simulink model "SimulationANTSMC"  (R2020b)
settings: Solver=ode3  StartTime=0.0  StopTime=100  FixedStep=0.001  RelTol=1e-6  EnableMultiTasking=on
model workspace (MAT data in the model file):
  time = 1
values from neighbouring files (symbols this model uses):
  beta = 2*x(3)/(1+x(3))    [GA_init.m]
  epstar = x(9)    [GA_init.m]
  g0 = x(5)    [GA_init.m]
  g1 = x(6)    [GA_init.m]
  g2 = x(7)    [GA_init.m]
  g3 = x(8)    [GA_init.m]
  gamma = x(3)    [GA_init.m]
  kappa = x(11)    [GA_init.m]
  landa = x(1)    [GA_init.m]
  nu = x(2)    [GA_init.m]
  vu = x(4)    [GA_init.m]
(part 9 of 18)

== matlab function SimulationANTSMC/Subsystem/System Dynamics ==
  data: disturbance output; u input; thetadot input; theta input; t input; y output
function [disturbance,y] = fcn(u,thetadot,theta,t)

theta1=theta(1);
theta2=theta(2);
theta3=theta(3);
theta4=theta(4);
theta5=theta(5);
theta6=theta(6);

thetadot1=thetadot(1);
thetadot2=thetadot(2);
thetadot3=thetadot(3);
thetadot4=thetadot(4);
thetadot5=thetadot(5);
thetadot6=thetadot(6);


MM =[ 0.1*cos(theta2 + theta3)^2 + (0.6*cos(theta2)*cos(theta4)*cos(theta6) + 0.2*cos(theta2)*cos(theta5)*sin(theta3) + 0.2*cos(theta3)*cos(theta5)*sin(theta2) + 1.5*cos(theta2)*cos(theta3)*cos(theta4)*cos(theta6) + 0.2*cos(theta2)*cos(theta3)*cos(theta4)*sin(theta5) + 1.4*cos(theta2)*cos(theta3)*sin(theta4)*sin(theta6) - 1.5*cos(theta4)*cos(theta6)*sin(theta2)*sin(theta3) + 1.4*cos(theta2)*cos(theta6)*sin(theta3)*sin(theta5) + 1.4*cos(theta3)*cos(theta6)*sin(theta2)*sin(theta5) - 0.6*cos(theta2)*cos(theta5)*sin(theta4)*sin(theta6) - 0.2*cos(theta4)*sin(theta2)*sin(theta3)*sin(theta5) - 1.4*sin(theta2)*sin(theta3)*sin(theta4)*sin(theta6) - 1.4*cos(theta2)*cos(theta3)*cos(theta4)*cos(theta5)*cos(theta6) - 1.5*cos(theta2)*cos(theta3)*cos(theta5)*sin(theta4)*sin(theta6) + 1.4*cos(theta4)*cos(theta5)*cos(theta6)*sin(theta2)*sin(theta3) + 1.5*cos(theta5)*sin(theta2)*sin(theta3)*sin(theta4)*sin(theta6))^2 + 0.101*sin(theta2 + theta3)^2 + (0.2*cos(theta6)*sin(theta2)*sin(theta3)*sin(theta4) - 0.2*cos(theta2)*cos(theta3)*cos(theta6)*sin(theta4) - 1.5*cos(theta2)*cos(theta3)*sin(theta4)*sin(theta5) - 0.6*cos(theta2)*sin(theta4)*sin(theta5) + 0.2*cos(theta2)*sin(theta3)*sin(theta5)*sin(theta6) + 0.2*cos(theta3)*sin(theta2)*sin(theta5)*sin(theta6) + 1.5*sin(theta2)*sin(theta3)*sin(theta4)*sin(theta5) - 0.2*cos(theta2)*cos(theta3)*cos(theta4)*cos(theta5)*sin(theta6) + 0.2*cos(theta4)*cos(theta5)*sin(theta2)*sin(theta3)*sin(theta6))^2 + (0.6*cos(theta2)*cos(theta4) - 1.5*cos(theta4)*sin(theta2)*sin(theta3) + 1.4*cos(theta2)*sin(theta3)*sin(theta5) + 1.4*cos(theta3)*sin(theta2)*sin(theta5) + 1.5*cos(theta2)*cos(theta3)*cos(theta4) + 0.2*cos(theta2)*cos(theta5)*sin(theta3) + 0.2*cos(theta3)*cos(theta5)*sin(theta2) - 1.4*cos(theta2)*cos(theta3)*cos(theta4)*cos(theta5) + 0.2*cos(theta2)*cos(theta3)*cos(theta4)*sin(theta5) + 1.4*cos(theta4)*cos(theta5)*sin(theta2)*sin(theta3) - 0.2*cos(theta4)*sin(theta2)*sin(theta3)*sin(theta5))^2 + (0.0001*cos(theta6)*sin(theta2)*sin(theta3)*sin(theta4) - 0.0001*cos(theta2)*cos(theta3)*cos(theta6)*sin(theta4) + 0.0001*cos(theta2)*sin(theta3)*sin(theta5)*sin(theta6) + 0.0001*cos(theta3)*sin(theta2)*sin(theta5)*sin(theta6) - 0.0001*cos(theta2)*cos(theta3)*cos(theta4)*cos(theta5)*sin(theta6) + 0.0001*cos(theta4)*cos(theta5)*sin(theta2)*sin(theta3)*sin(theta6))*(cos(theta6)*sin(theta2)*sin(theta3)*sin(theta4) - 1.0*cos(theta2)*cos(theta3)*cos(theta6)*sin(theta4) + cos(theta2)*sin(theta3)*sin(theta5)*sin(theta6) + cos(theta3)*sin(theta2)*sin(theta5)*sin(theta6) - 1.0*cos(theta2)*cos(theta3)*cos(theta4)*cos(theta5)*sin(theta6) + cos(theta4)*cos(theta5)*sin(theta2)*sin(theta3)*sin(theta6)) + (0.44721359549995793928183473374626*cos(theta2 + theta3 + 0.46364760900080611621425623146121) - 0.6*cos(theta2))^2 + 0.1*cos(theta2)^2 + 0.14*sin(theta2)^2 + (cos(theta2)*cos(theta5)*sin(theta3) + cos(theta3)*cos(theta5)*sin(theta2) + cos(theta2)*cos(theta3)*cos(theta4)*sin(theta5) - 1.0*cos(theta4)*sin(theta2)*sin(theta3)*sin(theta5))*(0.0001*cos(theta2)*cos(theta5)*sin(theta3) + 0.0001*cos(theta3)*cos(theta5)*sin(theta2) + 0.0001*cos(theta2)*cos(theta3)*cos(theta4)*sin(theta5) - 0.0001*cos(theta4)*sin(theta2)*sin(theta3)*sin(theta5)) + 0.01*sin(theta4)^2*(2.0*cos(theta2)*cos(theta3) + 6.0*cos(theta2)*sin(theta5) - 2.0*sin(theta2)*sin(theta3) - 15.0*sin(theta2)*sin(theta3)*sin(theta5) + 15.0*cos(theta2)*cos(theta3)*sin(theta5))^2 + 0.001*cos(theta2 + theta3)^2*cos(theta4)^2 + 0.01*sin(theta4)^2*(cos(theta2 + theta3) - 6.0*cos(theta2))^2 + 0.0415*cos(theta2 + theta3)^2*sin(theta4)^2 + (0.0005*cos(theta2)*cos(theta5)*sin(theta3) + 0.0005*cos(theta3)*cos(theta5)*sin(theta2) + 0.0005*cos(theta2)*cos(theta3)*cos(theta4)*sin(theta5) - 0.0005*cos(theta4)*sin(theta2)*sin(theta3)*sin(theta5))*(cos(theta2)*cos(theta5)*sin(theta3) + cos(theta3)*cos(theta5)*sin(theta2) + cos(theta2)*cos(theta3)*cos(theta4)*sin(theta5) - 1.0*cos(theta4)*sin(theta2)*sin(theta3)*sin(theta5)) + (0.0005*cos(theta2)*sin(theta3)*sin(theta5) + 0.0005*cos(theta3)*sin(theta2)*sin(theta5) - 0.0005*cos(theta2)*cos(theta3)*cos(theta4)*cos(theta5) + 0.0005*cos(theta4)*cos(theta5)*sin(theta2)*sin(theta3))*(cos(theta2)*sin(theta3)*sin(theta5) + cos(theta3)*sin(theta2)*sin(theta5) - 1.0*cos(theta2)*cos(theta3)*cos(theta4)*cos(theta5) + cos(theta4)*cos(theta5)*sin(theta2)*sin(theta3)) + 0.01*sin(theta4)^2*(6.0*cos(theta2)*cos(theta5) - 14.0*cos(theta2)*cos(theta3) + 14.0*sin(theta2)*sin(theta3) - 15.0*cos(theta5)*sin(theta2)*sin(theta3) + 15.0*cos(theta2)*cos(theta3)*cos(theta5))^2 + (0.6*cos(theta2)*cos(theta4) + 0.2*cos(theta2)*sin(theta3) + 0.2*cos(theta3)*sin(theta2) + 0.1*cos(theta4)*sin(theta2)*sin(theta3) - 0.1*cos(theta2)*cos(theta3)*cos(theta4))^2 + (0.0001*cos(theta2)*cos(theta3)*sin(theta4)*sin(theta6) + 0.0001*cos(theta2)*cos(theta6)*sin(theta3)*sin(theta5) + 0.0001*cos(theta3)*cos(theta6)*sin(theta2)*sin(theta5) - 0.0001*sin(theta2)*sin(theta3)*sin(theta4)*sin(theta6) - 0.0001*cos(theta2)*cos(theta3)*cos(theta4)*cos(theta5)*cos(theta6) + 0.0001*cos(theta4)*cos(theta5)*cos(theta6)*sin(theta2)*sin(theta3))*(cos(theta2)*cos(theta3)*sin(theta4)*sin(theta6) + cos(theta2)*cos(theta6)*sin(theta3)*sin(theta5) + cos(theta3)*cos(theta6)*sin(theta2)*sin(theta5) - 1.0*sin(theta2)*sin(theta3)*sin(theta4)*sin(theta6) - 1.0*cos(theta2)*cos(theta3)*cos(theta4)*cos(theta5)*cos(theta6) + cos(theta4)*cos(theta5)*cos(theta6)*sin(theta2)*sin(theta3)) + (0.6*cos(theta2)*cos(theta4)*sin(theta6) + 1.5*cos(theta2)*cos(theta3)*cos(theta4)*sin(theta6) - 1.4*cos(theta2)*cos(theta3)*cos(theta6)*sin(theta4) + 0.6*cos(theta2)*cos(theta5)*cos(theta6)*sin(theta4) - 1.5*cos(theta4)*sin(theta2)*sin(theta3)*sin(theta6) + 1.4*cos(theta6)*sin(theta2)*sin(theta3)*sin(theta4) + 1.4*cos(theta2)*sin(theta3)*sin(theta5)*sin(theta6) + 1.4*cos(theta3)*sin(theta2)*sin(theta5)*sin(theta6) - 1.4*cos(theta2)*cos(theta3)*cos(theta4)*cos(theta5)*sin(theta6) + 1.5*cos(theta2)*cos(theta3)*cos(theta5)*cos(theta6)*sin(theta4) + 1.4*cos(theta4)*cos(theta5)*sin(theta2)*sin(theta3)*sin(theta6) - 1.5*cos(theta5)*cos(theta6)*sin(theta2)*sin(theta3)*sin(theta4))^2 + 0.1, 0.12*sin(theta2)*sin(theta4) + 0.26*cos(theta2)*sin(theta3)*sin(theta4) + 0.26*cos(theta3)*sin(theta2)*sin(theta4) + 0.12*cos(theta5)*sin(theta2)*sin(theta4) + 0.12*cos(theta4)*sin(theta2)*sin(theta6) + 1.68*sin(theta2)*sin(theta4)*sin(theta5) - 0.56*cos(theta2)*cos(theta5)^2*sin(theta3)*sin(theta4) - 0.56*cos(theta3)*cos(theta5)^2*sin(theta2)*sin(theta4) - 3.92*cos(theta2)*cos(theta3)*cos(theta4)*sin(theta4) + 0.3*cos(theta2)*cos(theta5)*sin(theta3)*sin(theta4) + 0.3*cos(theta3)*cos(theta5)*sin(theta2)*sin(theta4) + 0.3*cos(theta2)*cos(theta4)*sin(theta3)*sin(theta6) + 0.28*cos(theta2)*cos(theta6)*sin(theta3)*sin(theta4) + 0.3*cos(theta3)*cos(theta4)*sin(theta2)*sin(theta6) + 0.28*cos(theta3)*cos(theta6)*sin(theta2)*sin(theta4) + 0.28*cos(theta2)*cos(theta3)*sin(theta5)*sin(theta6) + 0.12*cos(theta5)*cos(theta6)*sin(theta2)*sin(theta4) + 3.92*cos(theta4)*sin(theta2)*sin(theta3)*sin(theta4) + 4.2*cos(theta2)*sin(theta3)*sin(theta4)*sin(theta5) + 4.2*cos(theta3)*sin(theta2)*sin(theta4)*sin(theta5) - 0.28*sin(theta2)*sin(theta3)*sin(theta5)*sin(theta6) + 3.88*cos(theta2)*cos(theta3)*cos(theta4)*cos(theta5)^2*sin(theta4) - 0.04*cos(theta2)*cos(theta3)*cos(theta4)*cos(theta6)^2*sin(theta4) - 0.56*cos(theta2)*cos(theta3)*cos(theta4)^2*sin(theta5)*sin(theta6) - 0.56*cos(theta2)*cos(theta5)^2*cos(theta6)*sin(theta3)*sin(theta4) - 0.56*cos(theta3)*cos(theta5)^2*cos(theta6)*sin(theta2)*sin(theta4) - 3.88*cos(theta4)*cos(theta5)^2*sin(theta2)*sin(theta3)*sin(theta4) + 0.04*cos(theta4)*cos(theta6)^2*sin(theta2)*sin(theta3)*sin(theta4) + 0.56*cos(theta4)^2*sin(theta2)*sin(theta3)*sin(theta5)*sin(theta6) + 0.04*cos(theta2)*cos(theta3)*cos(theta5)*cos(theta6)*sin(theta6) - 0.28*cos(theta2)*cos(theta4)*cos(theta5)*sin(theta3)*sin(theta6) + 0.3*cos(theta2)*cos(theta5)*cos(theta6)*sin(theta3)*sin(theta4) - 0.28*cos(theta3)*cos(theta4)*cos(theta5)*sin(theta2)*sin(theta6) + 0.3*cos(theta3)*cos(theta5)*cos(theta6)*sin(theta2)*sin(theta4) - 3.88*cos(theta2)*cos(theta5)*sin(theta3)*sin(theta4)*sin(theta5) - 3.88*cos(theta3)*cos(theta5)*sin(theta2)*sin(theta4)*sin(theta5) - 0.04*cos(theta5)*cos(theta6)*sin(theta2)*sin(theta3)*sin(theta6) - 0.04*cos(theta2)*cos(theta3)*cos(theta4)*cos(theta5)^2*cos(theta6)^2*sin(theta4) + 0.04*cos(theta4)*cos(theta5)^2*cos(theta6)^2*sin(theta2)*sin(theta3)*sin(theta4) - 0.56*cos(theta2)*cos(theta3)*cos(theta4)*cos(theta5)*sin(theta4)*sin(theta5) + 0.04*cos(theta2)*cos(theta4)*cos(theta6)*sin(theta3)*sin(theta5)*sin(theta6) + 0.04*cos(theta3)*cos(theta4)*cos(theta6)*sin(theta2)*sin(theta5)*sin(theta6) + 0.56*cos(theta4)*cos(theta5)*sin(theta2)*sin(theta3)*sin(theta4)*sin(theta5) - 0.08*cos(theta2)*cos(theta3)*cos(theta4)^2*cos(theta5)*cos(theta6)*sin(theta6) + 0.04*cos(theta2)*cos(theta5)*cos(theta6)^2*sin(theta3)*sin(theta4)*sin(theta5) + 0.04*cos(theta3)*cos(theta5)*cos(theta6)^2*sin(theta2)*sin(theta4)*sin(theta5) + 0.08*cos(theta4)^2*cos(theta5)*cos(theta6)*sin(theta2)*sin(theta3)*sin(theta6) - 0.56*cos(theta2)*cos(theta3)*cos(theta4)*cos(theta5)*cos(theta6)*sin(theta4)*sin(theta5) + 0.56*cos(theta4)*cos(theta5)*cos(theta6)*sin(theta2)*sin(theta3)*sin(theta4)*sin(theta5), 0.26*cos(theta2)*sin(theta3)*sin(theta4) + 0.26*cos(theta3)*sin(theta2)*sin(theta4) - 0.56*cos(theta2)*cos(theta5)^2*sin(theta3)*sin(theta4) - 0.56*cos(theta3)*cos(theta5)^2*sin(theta2)*sin(theta4) - 3.92*cos(theta2)*cos(theta3)*cos(theta4)*sin(theta4) + 0.3*cos(theta2)*cos(theta5)*sin(theta3)*sin(theta4) + 0.3*cos(theta3)*cos(theta5)*sin(theta2)*sin(theta4) + 0.3*cos(theta2)*cos(theta4)*sin(theta3)*sin(theta6) + 0.28*cos(theta2)*cos(theta6)*sin(theta3)*sin(theta4) + 0.3*cos(theta3)*cos(theta4)*sin(theta2)*sin(theta6) + 0.28*cos(theta3)*cos(theta6)*sin(theta2)*sin(theta4) + 0.28*cos(theta2)*cos(theta3)*sin(theta5)*sin(theta6) + 3.92*cos(theta4)*sin(theta2)*sin(theta3)*sin(theta4) + 4.2*cos(theta2)*sin(theta3)*sin(theta4)*sin(theta5) + 4.2*cos(theta3)*sin(theta2)*sin(theta4)*sin(theta5) - 0.28*sin(theta2)*sin(theta3)*sin(theta5)*sin(theta6) + 3.88*cos(theta2)*cos(theta3)*cos(theta4)*cos(theta5)^2*sin(theta4) - 0.04*cos(theta2)*cos(theta3)*cos(theta4)*cos(theta6)^2*sin(theta4) - 0.56*cos(theta2)*cos(theta3)*cos(theta4)^2*sin(theta5)*sin(theta6) - 0.56*cos(theta2)*cos(theta5)^2*cos(theta6)*sin(theta3)*sin(theta4) - 0.56*cos(theta3)*cos(theta5)^2*cos(theta6)*sin(theta2)*sin(theta4) - 3.88*cos(theta4)*cos(theta5)^2*sin(theta2)*sin(theta3)*sin(theta4) + 0.04*cos(theta4)*cos(theta6)^2*sin(theta2)*sin(theta3)*sin(theta4) + 0.56*cos(theta4)^2*sin(theta2)*sin(theta3)*sin(theta5)*sin(theta6) + 0.04*cos(theta2)*cos(theta3)*cos(theta5)*cos(theta6)*sin(theta6) - 0.28*cos(theta2)*cos(theta4)*cos(theta5)*sin(theta3)*sin(theta6) + 0.3*cos(theta2)*cos(theta5)*cos(theta6)*sin(theta3)*sin(theta4) - 0.28*cos(theta3)*cos(theta4)*cos(theta5)*sin(theta2)*sin(theta6) + 0.3*cos(theta3)*cos(theta5)*cos(theta6)*sin(theta2)*sin(theta4) - 3.88*cos(theta2)*cos(theta5)*sin(theta3)*sin(theta4)*sin(theta5) - 3.88*cos(theta3)*cos(theta5)*sin(theta2)*sin(theta4)*sin(theta5) - 0.04*cos(theta5)*cos(theta6)*sin(theta2)*sin(theta3)*sin(theta6) - 0.04*cos(theta2)*cos(theta3)*cos(theta4)*cos(theta5)^2*cos(theta6)^2*sin(theta4) + 0.04*cos(theta4)*cos(theta5)^2*cos(theta6)^2*sin(theta2)*sin(theta3)*sin(theta4) - 0.56*cos(theta2)*cos(theta3)*cos(theta4)*cos(theta5)*sin(theta4)*sin(theta5) + 0.04*cos(theta2)*cos(theta4)*cos(theta6)*sin(theta3)*sin(theta5)*sin(theta6) + 0.04*cos(theta3)*cos(theta4)*cos(theta6)*sin(theta2)*sin(theta5)*sin(theta6) + 0.56*cos(theta4)*cos(theta5)*sin(theta2)*sin(theta3)*sin(theta4)*sin(theta5) - 0.08*cos(theta2)*cos(theta3)*cos(theta4)^2*cos(theta5)*cos(theta6)*sin(theta6) + 0.04*cos(theta2)*cos(theta5)*cos(theta6)^2*sin(theta3)*sin(theta4)*sin(theta5) + 0.04*cos(theta3)*cos(theta5)*cos(theta6)^2*sin(theta2)*sin(theta4)*sin(theta5) + 0.08*cos(theta4)^2*cos(theta5)*cos(theta6)*sin(theta2)*sin(theta3)*sin(theta6) - 0.56*cos(theta2)*cos(theta3)*cos(theta4)*cos(theta5)*cos(theta6)*sin(theta4)*sin(theta5) + 0.56*cos(theta4)*cos(theta5)*cos(theta6)*sin(theta2)*sin(theta3)*sin(theta4)*sin(theta5), 0.12*cos(theta2)*cos(theta4) + 4.0016*cos(theta2)*sin(theta3) + 4.0016*cos(theta3)*sin(theta2) - 0.26*cos(theta4)*sin(theta2)*sin(theta3) - 0.12*cos(theta2)*sin(theta4)*sin(theta6) - 3.88*cos(theta2)*cos(theta5)^2*sin(theta3) - 3.88*cos(theta3)*cos(theta5)^2*sin(theta2) - 0.04*cos(theta2)*cos(theta6)^2*sin(theta3) - 0.04*cos(theta3)*cos(theta6)^2*sin(theta2) + 0.26*cos(theta2)*cos(theta3)*cos(theta4) + 0.12*cos(theta2)*cos(theta4)*cos(theta5) + 1.68*cos(theta2)*cos(theta4)*sin(theta5) - 0.56*cos(theta2)*cos(theta3)*cos(theta4)*cos(theta5)^2 + 0.56*cos(theta4)*cos(theta5)^2*sin(theta2)*sin(theta3) + 0.04*cos(theta2)*cos(theta5)^2*cos(theta6)^2*sin(theta3) + 0.04*cos(theta3)*cos(theta5)^2*cos(theta6)^2*sin(theta2) + 0.3*cos(theta2)*cos(theta3)*cos(theta4)*cos(theta5) + 0.28*cos(theta2)*cos(theta3)*cos(theta4)*cos(theta6) + 0.12*cos(theta2)*cos(theta4)*cos(theta5)*cos(theta6) + 4.2*cos(theta2)*cos(theta3)*cos(theta4)*sin(theta5) - 0.3*cos(theta4)*cos(theta5)*sin(theta2)*sin(theta3) - 0.3*cos(theta2)*cos(theta3)*sin(theta4)*sin(theta6) + 0.56*cos(theta2)*cos(theta5)*sin(theta3)*sin(theta5) + 0.56*cos(theta3)*cos(theta5)*sin(theta2)*sin(theta5) - 0.28*cos(theta4)*cos(theta6)*sin(theta2)*sin(theta3) - 4.2*cos(theta4)*sin(theta2)*sin(theta3)*sin(theta5) + 0.3*sin(theta2)*sin(theta3)*sin(theta4)*sin(theta6) + 0.56*cos(theta4)*cos(theta5)^2*cos(theta6)*sin(theta2)*sin(theta3) + 0.3*cos(theta2)*cos(theta3)*cos(theta4)*cos(theta5)*cos(theta6) - 3.88*cos(theta2)*cos(theta3)*cos(theta4)*cos(theta5)*sin(theta5) + 0.28*cos(theta2)*cos(theta3)*cos(theta5)*sin(theta4)*sin(theta6) - 0.3*cos(theta4)*cos(theta5)*cos(theta6)*sin(theta2)*sin(theta3) + 0.56*cos(theta2)*cos(theta5)*cos(theta6)*sin(theta3)*sin(theta5) + 0.56*cos(theta3)*cos(theta5)*cos(theta6)*sin(theta2)*sin(theta5) + 3.88*cos(theta4)*cos(theta5)*sin(theta2)*sin(theta3)*sin(theta5) - 0.28*cos(theta5)*sin(theta2)*sin(theta3)*sin(theta4)*sin(theta6) - 0.56*cos(theta2)*cos(theta3)*cos(theta4)*cos(theta5)^2*cos(theta6) - 0.04*cos(theta2)*cos(theta3)*cos(theta6)*sin(theta4)*sin(theta5)*sin(theta6) + 0.04*cos(theta6)*sin(theta2)*sin(theta3)*sin(theta4)*sin(theta5)*sin(theta6) + 0.04*cos(theta2)*cos(theta3)*cos(theta4)*cos(theta5)*cos(theta6)^2*sin(theta5) - 0.04*cos(theta4)*cos(theta5)*cos(theta6)^2*sin(theta2)*sin(theta3)*sin(theta5), 3.9606*sin(theta2)*sin(theta3)*sin(theta4) - 0.12*cos(theta2)*sin(theta4)*sin(theta5) - 3.9606*cos(theta2)*cos(theta3)*sin(theta4) + 1.68*cos(theta2)*cos(theta5)*sin(theta4) - 0.04*cos(theta2)*cos(theta3)*cos(theta6)^2*sin(theta4) + 0.04*cos(theta6)^2*sin(theta2)*sin(theta3)*sin(theta4) + 4.2*cos(theta2)*cos(theta3)*cos(theta5)*sin(theta4) - 0.3*cos(theta2)*cos(theta3)*sin(theta4)*sin(theta5) - 0.28*cos(theta2)*cos(theta5)*sin(theta3)*sin(theta6) - 0.28*cos(theta3)*cos(theta5)*sin(theta2)*sin(theta6) - 0.12*cos(theta2)*cos(theta6)*sin(theta4)*sin(theta5) - 4.2*cos(theta5)*sin(theta2)*sin(theta3)*sin(theta4) + 0.3*sin(theta2)*sin(theta3)*sin(theta4)*sin(theta5) - 0.28*cos(theta2)*cos(theta3)*cos(theta4)*sin(theta5)*sin(theta6) - 0.3*cos(theta2)*cos(theta3)*cos(theta6)*sin(theta4)*sin(theta5) + 0.04*cos(theta2)*cos(theta6)*sin(theta3)*sin(theta5)*sin(theta6) + 0.04*cos(theta3)*cos(theta6)*sin(theta2)*sin(theta5)*sin(theta6) + 0.28*cos(theta4)*sin(theta2)*sin(theta3)*sin(theta5)*sin(theta6) + 0.3*cos(theta6)*sin(theta2)*sin(theta3)*sin(theta4)*sin(theta5) - 0.04*cos(theta2)*cos(theta3)*cos(theta4)*cos(theta5)*cos(theta6)*sin(theta6) + 0.04*cos(theta4)*cos(theta5)*cos(theta6)*sin(theta2)*sin(theta3)*sin(theta6), 0.12*cos(theta2)*cos(theta4)*cos(theta6) + 0.0401*cos(theta2)*cos(theta5)*sin(theta3) + 0.0401*cos(theta3)*cos(theta5)*sin(theta2) + 0.3*cos(theta2)*cos(theta3)*cos(theta4)*cos(theta6) + 0.0401*cos(theta2)*cos(theta3)*cos(theta4)*sin(theta5) + 0.28*cos(theta2)*cos(theta3)*sin(theta4)*sin(theta6) - 0.3*cos(theta4)*cos(theta6)*sin(theta2)*sin(theta3) + 0.28*cos(theta2)*cos(theta6)*sin(theta3)*sin(theta5) + 0.28*cos(theta3)*cos(theta6)*sin(theta2)*sin(theta5) - 0.12*cos(theta2)*cos(theta5)*sin(theta4)*sin(theta6) - 0.0401*cos(theta4)*sin(theta2)*sin(theta3)*sin(theta5) - 0.28*sin(theta2)*sin(theta3)*sin(theta4)*sin(theta6) - 0.28*cos(theta2)*cos(theta3)*cos(theta4)*cos(theta5)*cos(theta6) - 0.3*cos(theta2)*cos(theta3)*cos(theta5)*sin(theta4)*sin(theta6) + 0.28*cos(theta4)*cos(theta5)*cos(theta6)*sin(theta2)*sin(theta3) + 0.3*cos(theta5)*sin(theta2)*sin(theta3)*sin(theta4)*sin(theta6);
                                                                                                                                                                                                                                                                                                                                                                                                                                                                                                                                                                                                                                                                                                                                                                                                                                                                                                                                                                                                                                                                                                                                                                                                                                                                                                                                                                                                                                                                                                                                                                                                                                                                                                                                                                                                                                                                                                                                                                                                                                                                                                                                                                                                                                                                                                                                                                                                                                                                                                                                                                                                                                                                                                                                                                                                                                                                                                                                                                                                                                                                0.12*sin(theta2)*sin(theta4) + 0.26*cos(theta2)*sin(theta3)*sin(theta4) + 0.26*cos(theta3)*sin(theta2)*sin(theta4) + 0.12*cos(theta5)*sin(theta2)*sin(theta4) + 0.12*cos(theta4)*sin(theta2)*sin(theta6) + 1.68*sin(theta2)*sin(theta4)*sin(theta5) - 0.56*cos(theta2)*cos(theta5)^2*sin(theta3)*sin(theta4) - 0.56*cos(theta3)*cos(theta5)^2*sin(theta2)*sin(theta4) - 3.92*cos(theta2)*cos(theta3)*cos(theta4)*sin(theta4) + 0.3*cos(theta2)*cos(theta5)*sin(theta3)*sin(theta4) + 0.3*cos(theta3)*cos(theta5)*sin(theta2)*sin(theta4) + 0.3*cos(theta2)*cos(theta4)*sin(theta3)*sin(theta6) + 0.28*cos(theta2)*cos(theta6)*sin(theta3)*sin(theta4) + 0.3*cos(theta3)*cos(theta4)*sin(theta2)*sin(theta6) + 0.28*cos(theta3)*cos(theta6)*sin(theta2)*sin(theta4) + 0.28*cos(theta2)*cos(theta3)*sin(theta5)*sin(theta6) + 0.12*cos(theta5)*cos(theta6)*sin(theta2)*sin(theta4) + 3.92*cos(theta4)*sin(theta2)*sin(theta3)*sin(theta4) + 4.2*cos(theta2)*sin(theta3)*sin(theta4)*sin(theta5) + 4.2*cos(theta3)*sin(theta2)*sin(theta4)*sin(theta5) - 0.28*sin(theta2)*sin(theta3)*sin(theta5)*sin(theta6) + 3.88*cos(theta2)*cos(theta3)*cos(theta4)*cos(theta5)^2*sin(theta4) - 0.04*cos(theta2)*cos(theta3)*cos(theta4)*cos(theta6)^2*sin(theta4) - 0.56*cos(theta2)*cos(theta3)*cos(theta4)^2*sin(theta5)*sin(theta6) - 0.56*cos(theta2)*cos(theta5)^2*cos(theta6)*sin(theta3)*sin(theta4) - 0.56*cos(theta3)*cos(theta5)^2*cos(theta6)*sin(theta2)*sin(theta4) - 3.88*cos(theta4)*cos(theta5)^2*sin(theta2)*sin(theta3)*sin(theta4) + 0.04*cos(theta4)*cos(theta6)^2*sin(theta2)*sin(theta3)*sin(theta4) + 0.56*cos(theta4)^2*sin(theta2)*sin(theta3)*sin(theta5)*sin(theta6) + 0.04*cos(theta2)*cos(theta3)*cos(theta5)*cos(theta6)*sin(theta6) - 0.28*cos(theta2)*cos(theta4)*cos(theta5)*sin(theta3)*sin(theta6) + 0.3*cos(theta2)*cos(theta5)*cos(theta6)*sin(theta3)*sin(theta4) - 0.28*cos(theta3)*cos(theta4)*cos(theta5)*sin(theta2)*sin(theta6) + 0.3*cos(theta3)*cos(theta5)*cos(theta6)*sin(theta2)*sin(theta4) - 3.88*cos(theta2)*cos(theta5)*sin(theta3)*sin(theta4)*sin(theta5) - 3.88*cos(theta3)*cos(theta5)*sin(theta2)*sin(theta4)*sin(theta5) - 0.04*cos(theta5)*cos(theta6)*sin(theta2)*sin(theta3)*sin(theta6) - 0.04*cos(theta2)*cos(theta3)*cos(theta4)*cos(theta5)^2*cos(theta6)^2*sin(theta4) + 0.04*cos(theta4)*cos(theta5)^2*cos(theta6)^2*sin(theta2)*sin(theta3)*sin(theta4) - 0.56*cos(theta2)*cos(theta3)*cos(theta4)*cos(theta5)*sin(theta4)*sin(theta5) + 0.04*cos(theta2)*cos(theta4)*cos(theta6)*sin(theta3)*sin(theta5)*sin(theta6) + 0.04*cos(theta3)*cos(theta4)*cos(theta6)*sin(theta2)*sin(theta5)*sin(theta6) + 0.56*cos(theta4)*cos(theta5)*sin(theta2)*sin(theta3)*sin(theta4)*sin(theta5) - 0.08*cos(theta2)*cos(theta3)*cos(theta4)^2*cos(theta5)*cos(theta6)*sin(theta6) + 0.04*cos(theta2)*cos(theta5)*cos(theta6)^2*sin(theta3)*sin(theta4)*sin(theta5) + 0.04*cos(theta3)*cos(theta5)*cos(theta6)^2*sin(theta2)*sin(theta4)*sin(theta5) + 0.08*cos(theta4)^2*cos(theta5)*cos(theta6)*sin(theta2)*sin(theta3)*sin(theta6) - 0.56*cos(theta2)*cos(theta3)*cos(theta4)*cos(theta5)*cos(theta6)*sin(theta4)*sin(theta5) + 0.56*cos(theta4)*cos(theta5)*cos(theta6)*sin(theta2)*sin(theta3)*sin(theta4)*sin(theta5),                                                                                                                                                                                                                                                                                                                                                                                                                                                                                                                                                                                                                                                                                                                                                                                                                                                                                                                                                                                                                                                                                                                                                                                                                                                                                                                                                                                                                                                       0.9751025587085698956283164129538*cos(2.0*theta5 + 0.14407254065728860693496196531882) - 0.4875512793542849478141582064769*cos(2.0*theta5 - 2.0*theta4 + 0.14407254065728860693496196531882) - 0.4875512793542849478141582064769*cos(2.0*theta4 + 2.0*theta5 + 0.14407254065728860693496196531882) + 1.005*cos(2.0*theta4) + 0.005*cos(2.0*theta6) + 3.0*cos(theta3) - 8.4*cos(theta5) + 0.24*sin(theta3) + 0.6*sin(theta5) - 3.36*cos(theta3)*cos(theta5) + 0.24*cos(theta4)*sin(theta3) + 0.24*cos(theta3)*sin(theta5) - 3.6093362052733169452242541700662e-34*cos(theta5)*sin(theta3) + 0.6*cos(theta6)*sin(theta5) - 4.0425025303541333499165546182713e-33*sin(theta3)*sin(theta5) + 0.015*cos(2.0*theta4)*cos(2.0*theta6) - 0.005*cos(2.0*theta5)*cos(2.0*theta6) - 1.3775324423698681734008631295573e-40*cos(2.0*theta4)*cos(theta3) - 0.14*sin(2.0*theta5)*cos(theta6) - 2.6333865515596676711856401422974e-35*cos(theta3)*sin(theta4)*sin(theta5) + 3.36*cos(theta4)*sin(theta3)*sin(theta5) - 2.6333865515596676711856401422974e-35*cos(theta5)*sin(theta3)*sin(theta4) + 3.7972710287846561672182643666688e-35*sin(theta3)*sin(theta4)*sin(theta5) - 0.24*sin(theta3)*sin(theta4)*sin(theta6) + 0.14*cos(2.0*theta4)*sin(2.0*theta5)*cos(theta6) - 0.02*sin(2.0*theta4)*sin(2.0*theta6)*cos(theta5) - 0.28*sin(2.0*theta4)*sin(theta5)*sin(theta6) + 0.005*cos(2.0*theta4)*cos(2.0*theta5)*cos(2.0*theta6) + 2.6333865515596676711856401422974e-35*cos(theta3)*cos(theta4)*cos(theta5) - 3.7972710287846561672182643666688e-35*cos(theta3)*cos(theta4)*sin(theta5) - 3.7972710287846561672182643666688e-35*cos(theta3)*cos(theta5)*sin(theta4) + 0.24*cos(theta4)*cos(theta5)*sin(theta3) + 0.24*cos(theta3)*cos(theta6)*sin(theta5) + 0.24*cos(theta4)*cos(theta5)*cos(theta6)*sin(theta3) + 9.4066,                                                                                                                                                                                                                                                                                                                                                                                                                                                                                                                                                                                                                                                                                                                                                                                                                                                                                                                                                                                                                                                                                                                                                                                                                                                                                                                                                                                                                                                                                                                                                                                                                                                                                                                                                                                                                                                                                                                                                                                                                                                                                             1.5*cos(theta3) - 0.28*sin(2*theta5) - 8.4*cos(theta5) + 0.12*sin(theta3) + 0.6*sin(theta5) - 1.68*cos(theta3)*cos(theta5) + 0.12*cos(theta4)*sin(theta3) + 0.12*cos(theta3)*sin(theta5) + 0.6*cos(theta6)*sin(theta5) + 3.92*cos(theta4)^2 + 3.88*cos(theta5)^2 - 3.88*cos(theta4)^2*cos(theta5)^2 + 0.04*cos(theta4)^2*cos(theta6)^2 - 0.04*cos(theta5)^2*cos(theta6)^2 + 0.04*cos(theta4)^2*cos(theta5)^2*cos(theta6)^2 + 1.68*cos(theta4)*sin(theta3)*sin(theta5) - 0.12*sin(theta3)*sin(theta4)*sin(theta6) + 0.56*cos(theta4)^2*cos(theta5)*sin(theta5) + 0.12*cos(theta4)*cos(theta5)*sin(theta3) + 0.12*cos(theta3)*cos(theta6)*sin(theta5) - 0.56*cos(theta5)*cos(theta6)*sin(theta5) + 0.56*cos(theta4)^2*cos(theta5)*cos(theta6)*sin(theta5) + 0.12*cos(theta4)*cos(theta5)*cos(theta6)*sin(theta3) - 0.56*cos(theta4)*sin(theta4)*sin(theta5)*sin(theta6) - 0.08*cos(theta4)*cos(theta5)*cos(theta6)*sin(theta4)*sin(theta6) + 4.8916,                                                                                                                                                                                                                                                                                                                                                                                                                                                                                                                                                                                                                                                                                                                                                                                                                                                                                                                                                                                                                                                                                                                                                                                                                                                                                                                                                                                                                                                                                                                                                                                                        0.26*sin(theta4) + 0.12*cos(theta3)*sin(theta4) + 0.3*cos(theta5)*sin(theta4) + 0.3*cos(theta4)*sin(theta6) + 0.28*cos(theta6)*sin(theta4) + 4.2*sin(theta4)*sin(theta5) - 0.56*cos(theta5)^2*sin(theta4) + 1.68*cos(theta3)*sin(theta4)*sin(theta5) - 3.88*cos(theta5)*sin(theta4)*sin(theta5) - 0.56*cos(theta5)^2*cos(theta6)*sin(theta4) + 0.12*cos(theta3)*cos(theta5)*sin(theta4) + 0.12*cos(theta3)*cos(theta4)*sin(theta6) - 0.28*cos(theta4)*cos(theta5)*sin(theta6) + 0.3*cos(theta5)*cos(theta6)*sin(theta4) + 0.04*cos(theta5)*cos(theta6)^2*sin(theta4)*sin(theta5) + 0.12*cos(theta3)*cos(theta5)*cos(theta6)*sin(theta4) + 0.04*cos(theta4)*cos(theta6)*sin(theta5)*sin(theta6) - 7.346839692639296924804603357639e-40*cos(theta4)*cos(theta5)*cos(theta6)*sin(theta5)*sin(theta6),                                                                                                                                                                                                                                                                                                                                                                                                                                                                                                                                                                                                              3.9606*cos(theta4) - 4.2*cos(theta4)*cos(theta5) - 1.1479437019748901445007192746311e-41*cos(theta4)*cos(theta6) + 0.12*cos(theta5)*sin(theta3) + 0.3*cos(theta4)*sin(theta5) + 1.68*sin(theta3)*sin(theta5) + 0.04*cos(theta4)*cos(theta6)^2 + 1.1479437019748901445007192746311e-41*cos(theta5)*sin(theta4)*sin(theta6) - 0.28*sin(theta4)*sin(theta5)*sin(theta6) - 1.68*cos(theta3)*cos(theta4)*cos(theta5) + 0.12*cos(theta3)*cos(theta4)*sin(theta5) + 0.12*cos(theta5)*cos(theta6)*sin(theta3) + 0.3*cos(theta4)*cos(theta6)*sin(theta5) + 0.12*cos(theta3)*cos(theta4)*cos(theta6)*sin(theta5) - 0.04*cos(theta5)*cos(theta6)*sin(theta4)*sin(theta6),                                                                                                                                                                                                                                                                                                                                                                                                                                                                                                                                                                                                 0.3*cos(theta6)*sin(theta4) - 0.28*cos(theta4)*sin(theta6) + 0.0401*sin(theta4)*sin(theta5) - 0.12*sin(theta3)*sin(theta5)*sin(theta6) + 0.12*cos(theta3)*cos(theta6)*sin(theta4) + 0.3*cos(theta4)*cos(theta5)*sin(theta6) - 0.28*cos(theta5)*cos(theta6)*sin(theta4) + 0.12*cos(theta3)*cos(theta4)*cos(theta5)*sin(theta6);
                                                                                                                                                                                                                                                                                                                                                                                                                                                                                                                                                                                                                                                                                                                                                                                                                                                                                                                                                                                                                                                                                                                                                                                                                                                                                                                                                                                                                                                                                                                                                                                                                                                                                                                                                                                                                                                                                                                                                                                                                                                                                                                                                                                                                                                                                                                                                                                                                                                                                                                                                                                                                                                                                                                                                                                                                                                                                                                                                                                                                                                                                                                                                                                                                                                                                       0.26*cos(theta2)*sin(theta3)*sin(theta4) + 0.26*cos(theta3)*sin(theta2)*sin(theta4) - 0.56*cos(theta2)*cos(theta5)^2*sin(theta3)*sin(theta4) - 0.56*cos(theta3)*cos(theta5)^2*sin(theta2)*sin(theta4) - 3.92*cos(theta2)*cos(theta3)*cos(theta4)*sin(theta4) + 0.3*cos(theta2)*cos(theta5)*sin(theta3)*sin(theta4) + 0.3*cos(theta3)*cos(theta5)*sin(theta2)*sin(theta4) + 0.3*cos(theta2)*cos(theta4)*sin(theta3)*sin(theta6) + 0.28*cos(theta2)*cos(theta6)*sin(theta3)*sin(theta4) + 0.3*cos(theta3)*cos(theta4)*sin(theta2)*sin(theta6) + 0.28*cos(theta3)*cos(theta6)*sin(theta2)*sin(theta4) + 0.28*cos(theta2)*cos(theta3)*sin(theta5)*sin(theta6) + 3.92*cos(theta4)*sin(theta2)*sin(theta3)*sin(theta4) + 4.2*cos(theta2)*sin(theta3)*sin(theta4)*sin(theta5) + 4.2*cos(theta3)*sin(theta2)*sin(theta4)*sin(theta5) - 0.28*sin(theta2)*sin(theta3)*sin(theta5)*sin(theta6) + 3.88*cos(theta2)*cos(theta3)*cos(theta4)*cos(theta5)^2*sin(theta4) - 0.04*cos(theta2)*cos(theta3)*cos(theta4)*cos(theta6)^2*sin(theta4) - 0.56*cos(theta2)*cos(theta3)*cos(theta4)^2*sin(theta5)*sin(theta6) - 0.56*cos(theta2)*cos(theta5)^2*cos(theta6)*sin(theta3)*sin(theta4) - 0.56*cos(theta3)*cos(theta5)^2*cos(theta6)*sin(theta2)*sin(theta4) - 3.88*cos(theta4)*cos(theta5)^2*sin(theta2)*sin(theta3)*sin(theta4) + 0.04*cos(theta4)*cos(theta6)^2*sin(theta2)*sin(theta3)*sin(theta4) + 0.56*cos(theta4)^2*sin(theta2)*sin(theta3)*sin(theta5)*sin(theta6) + 0.04*cos(theta2)*cos(theta3)*cos(theta5)*cos(theta6)*sin(theta6) - 0.28*cos(theta2)*cos(theta4)*cos(theta5)*sin(theta3)*sin(theta6) + 0.3*cos(theta2)*cos(theta5)*cos(theta6)*sin(theta3)*sin(theta4) - 0.28*cos(theta3)*cos(theta4)*cos(theta5)*sin(theta2)*sin(theta6) + 0.3*cos(theta3)*cos(theta5)*cos(theta6)*sin(theta2)*sin(theta4) - 3.88*cos(theta2)*cos(theta5)*sin(theta3)*sin(theta4)*sin(theta5) - 3.88*cos(theta3)*cos(theta5)*sin(theta2)*sin(theta4)*sin(theta5) - 0.04*cos(theta5)*cos(theta6)*sin(theta2)*sin(theta3)*sin(theta6) - 0.04*cos(theta2)*cos(theta3)*cos(theta4)*cos(theta5)^2*cos(theta6)^2*sin(theta4) + 0.04*cos(theta4)*cos(theta5)^2*cos(theta6)^2*sin(theta2)*sin(theta3)*sin(theta4) - 0.56*cos(theta2)*cos(theta3)*cos(theta4)*cos(theta5)*sin(theta4)*sin(theta5) + 0.04*cos(theta2)*cos(theta4)*cos(theta6)*sin(theta3)*sin(theta5)*sin(theta6) + 0.04*cos(theta3)*cos(theta4)*cos(theta6)*sin(theta2)*sin(theta5)*sin(theta6) + 0.56*cos(theta4)*cos(theta5)*sin(theta2)*sin(theta3)*sin(theta4)*sin(theta5) - 0.08*cos(theta2)*cos(theta3)*cos(theta4)^2*cos(theta5)*cos(theta6)*sin(theta6) + 0.04*cos(theta2)*cos(theta5)*cos(theta6)^2*sin(theta3)*sin(theta4)*sin(theta5) + 0.04*cos(theta3)*cos(theta5)*cos(theta6)^2*sin(theta2)*sin(theta4)*sin(theta5) + 0.08*cos(theta4)^2*cos(theta5)*cos(theta6)*sin(theta2)*sin(theta3)*sin(theta6) - 0.56*cos(theta2)*cos(theta3)*cos(theta4)*cos(theta5)*cos(theta6)*sin(theta4)*sin(theta5) + 0.56*cos(theta4)*cos(theta5)*cos(theta6)*sin(theta2)*sin(theta3)*sin(theta4)*sin(theta5),                                                                                                                                                                                                                                                                                                                                                                                                                                                                                                                                                                                                                                                                                                                                                                                                                                                                                                                                                                                                                                                                                                                                                                                                                                                                                                                                                                                                                                                                                                                                                                                                                                                                                                                                                                                                                                                                                                                                                                                                                                                                                                                                                                                                                                                                                                                    1.5*cos(theta3) - 0.28*sin(2*theta5) - 8.4*cos(theta5) + 0.12*sin(theta3) + 0.6*sin(theta5) - 1.68*cos(theta3)*cos(theta5) + 0.12*cos(theta4)*sin(theta3) + 0.12*cos(theta3)*sin(theta5) + 0.6*cos(theta6)*sin(theta5) + 3.92*cos(theta4)^2 + 3.88*cos(theta5)^2 - 3.88*cos(theta4)^2*cos(theta5)^2 + 0.04*cos(theta4)^2*cos(theta6)^2 - 0.04*cos(theta5)^2*cos(theta6)^2 + 0.04*cos(theta4)^2*cos(theta5)^2*cos(theta6)^2 + 1.68*cos(theta4)*sin(theta3)*sin(theta5) - 0.12*sin(theta3)*sin(theta4)*sin(theta6) + 0.56*cos(theta4)^2*cos(theta5)*sin(theta5) + 0.12*cos(theta4)*cos(theta5)*sin(theta3) + 0.12*cos(theta3)*cos(theta6)*sin(theta5) - 0.56*cos(theta5)*cos(theta6)*sin(theta5) + 0.56*cos(theta4)^2*cos(theta5)*cos(theta6)*sin(theta5) + 0.12*cos(theta4)*cos(theta5)*cos(theta6)*sin(theta3) - 0.56*cos(theta4)*sin(theta4)*sin(theta5)*sin(theta6) - 0.08*cos(theta4)*cos(theta5)*cos(theta6)*sin(theta4)*sin(theta6) + 4.8916,                                                                                                                                                                                                                                                                                                                                                                                                                                                                                                                                                                                                                                                                                                                                                                                                                                                                                                                                                                                                                                                                                                                                                                                                                                                                                                                                                                                                                                                                                                                                                                                                                                                                                                                                                                                                                                                                                                                                                                                                                                                                                                                                                                                                                                                                                                                                                                                                                                                                  0.6*sin(theta5) - 8.4*cos(theta5) - 0.28*sin(2*theta5) + 0.6*cos(theta6)*sin(theta5) + 3.92*cos(theta4)^2 + 3.88*cos(theta5)^2 - 3.88*cos(theta4)^2*cos(theta5)^2 + 0.04*cos(theta4)^2*cos(theta6)^2 - 0.04*cos(theta5)^2*cos(theta6)^2 + 0.04*cos(theta4)^2*cos(theta5)^2*cos(theta6)^2 + 0.56*cos(theta4)^2*cos(theta5)*sin(theta5) - 0.56*cos(theta5)*cos(theta6)*sin(theta5) + 0.56*cos(theta4)^2*cos(theta5)*cos(theta6)*sin(theta5) - 0.56*cos(theta4)*sin(theta4)*sin(theta5)*sin(theta6) - 0.08*cos(theta4)*cos(theta5)*cos(theta6)*sin(theta4)*sin(theta6) + 4.8916,                                                                                                                                                                                                                                                                                                                                                                                                                                                                                                                                                                                                                                                                                                                                                                                                                                                                                                                                                                                                                                                                                                                                                                                                                                                                                                                                                                                                                                                                                                                                                                                                                                                                                                                                                                                                                               0.26*sin(theta4) + 0.3*cos(theta5)*sin(theta4) + 0.3*cos(theta4)*sin(theta6) + 0.28*cos(theta6)*sin(theta4) + 4.2*sin(theta4)*sin(theta5) - 0.56*cos(theta5)^2*sin(theta4) - 3.88*cos(theta5)*sin(theta4)*sin(theta5) - 0.56*cos(theta5)^2*cos(theta6)*sin(theta4) - 0.28*cos(theta4)*cos(theta5)*sin(theta6) + 0.3*cos(theta5)*cos(theta6)*sin(theta4) + 0.04*cos(theta5)*cos(theta6)^2*sin(theta4)*sin(theta5) + 0.04*cos(theta4)*cos(theta6)*sin(theta5)*sin(theta6) - 7.346839692639296924804603357639e-40*cos(theta4)*cos(theta5)*cos(theta6)*sin(theta5)*sin(theta6),                                                                                                                                                                                                                                                                                                                                                                                                                                                                                                                                                                                                                                                                                                                                                                                                                                                                    3.9606*cos(theta4) - 4.2*cos(theta4)*cos(theta5) - 1.1479437019748901445007192746311e-41*cos(theta4)*cos(theta6) + 0.3*cos(theta4)*sin(theta5) + 0.04*cos(theta4)*cos(theta6)^2 + 1.1479437019748901445007192746311e-41*cos(theta5)*sin(theta4)*sin(theta6) - 0.28*sin(theta4)*sin(theta5)*sin(theta6) + 0.3*cos(theta4)*cos(theta6)*sin(theta5) - 0.04*cos(theta5)*cos(theta6)*sin(theta4)*sin(theta6),                                                                                                                                                                                                                                                                                                                                                                                                                                                                                                                                                                                                                                                                                                                                              0.3*cos(theta6)*sin(theta4) - 0.28*cos(theta4)*sin(theta6) + 0.0401*sin(theta4)*sin(theta5) + 0.3*cos(theta4)*cos(theta5)*sin(theta6) - 0.28*cos(theta5)*cos(theta6)*sin(theta4);
                                                                                                                                                                                                                                                                                                                                                                                                                                                                                                                                                                                                                                                                                                                                                                                                                                                                                                                                                                                                                                                                                                                                                                                                                                                                                                                                                                                                                                                                                                                                                                                                                                                                                                                                                                                                                                                                                                                                                                                                                                                                                                                                                                                                                                                                                                                                                                                                                                                                                                                                                                                                                                                                                                                                                                                                                                                                                                                                                                                                                                                                                                                                                                                                                                                                                                                                                                                                                                                                                                                                                                                                                                                                                                                                                                                                                                                                                                                            0.12*cos(theta2)*cos(theta4) + 4.0016*cos(theta2)*sin(theta3) + 4.0016*cos(theta3)*sin(theta2) - 0.26*cos(theta4)*sin(theta2)*sin(theta3) - 0.12*cos(theta2)*sin(theta4)*sin(theta6) - 3.88*cos(theta2)*cos(theta5)^2*sin(theta3) - 3.88*cos(theta3)*cos(theta5)^2*sin(theta2) - 0.04*cos(theta2)*cos(theta6)^2*sin(theta3) - 0.04*cos(theta3)*cos(theta6)^2*sin(theta2) + 0.26*cos(theta2)*cos(theta3)*cos(theta4) + 0.12*cos(theta2)*cos(theta4)*cos(theta5) + 1.68*cos(theta2)*cos(theta4)*sin(theta5) - 0.56*cos(theta2)*cos(theta3)*cos(theta4)*cos(theta5)^2 + 0.56*cos(theta4)*cos(theta5)^2*sin(theta2)*sin(theta3) + 0.04*cos(theta2)*cos(theta5)^2*cos(theta6)^2*sin(theta3) + 0.04*cos(theta3)*cos(theta5)^2*cos(theta6)^2*sin(theta2) + 0.3*cos(theta2)*cos(theta3)*cos(theta4)*cos(theta5) + 0.28*cos(theta2)*cos(theta3)*cos(theta4)*cos(theta6) + 0.12*cos(theta2)*cos(theta4)*cos(theta5)*cos(theta6) + 4.2*cos(theta2)*cos(theta3)*cos(theta4)*sin(theta5) - 0.3*cos(theta4)*cos(theta5)*sin(theta2)*sin(theta3) - 0.3*cos(theta2)*cos(theta3)*sin(theta4)*sin(theta6) + 0.56*cos(theta2)*cos(theta5)*sin(theta3)*sin(theta5) + 0.56*cos(theta3)*cos(theta5)*sin(theta2)*sin(theta5) - 0.28*cos(theta4)*cos(theta6)*sin(theta2)*sin(theta3) - 4.2*cos(theta4)*sin(theta2)*sin(theta3)*sin(theta5) + 0.3*sin(theta2)*sin(theta3)*sin(theta4)*sin(theta6) + 0.56*cos(theta4)*cos(theta5)^2*cos(theta6)*sin(theta2)*sin(theta3) + 0.3*cos(theta2)*cos(theta3)*cos(theta4)*cos(theta5)*cos(theta6) - 3.88*cos(theta2)*cos(theta3)*cos(theta4)*cos(theta5)*sin(theta5) + 0.28*cos(theta2)*cos(theta3)*cos(theta5)*sin(theta4)*sin(theta6) - 0.3*cos(theta4)*cos(theta5)*cos(theta6)*sin(theta2)*sin(theta3) + 0.56*cos(theta2)*cos(theta5)*cos(theta6)*sin(theta3)*sin(theta5) + 0.56*cos(theta3)*cos(theta5)*cos(theta6)*sin(theta2)*sin(theta5) + 3.88*cos(theta4)*cos(theta5)*sin(theta2)*sin(theta3)*sin(theta5) - 0.28*cos(theta5)*sin(theta2)*sin(theta3)*sin(theta4)*sin(theta6) - 0.56*cos(theta2)*cos(theta3)*cos(theta4)*cos(theta5)^2*cos(theta6) - 0.04*cos(theta2)*cos(theta3)*cos(theta6)*sin(theta4)*sin(theta5)*sin(theta6) + 0.04*cos(theta6)*sin(theta2)*sin(theta3)*sin(theta4)*sin(theta5)*sin(theta6) + 0.04*cos(theta2)*cos(theta3)*cos(theta4)*cos(theta5)*cos(theta6)^2*sin(theta5) - 0.04*cos(theta4)*cos(theta5)*cos(theta6)^2*sin(theta2)*sin(theta3)*sin(theta5),                                                                                                                                                                                                                                                                                                                                                                                                                                                                                                                                                                                                                                                                                                                                                                                                                                                                                                                                                                                                                                                                                                                                                                                                                                                                                                                                                                                                                                                                                                                                                                                                                                                                                                                                                                                                                                                                                                                                                                                                                                                                                                                                                                                                                                                                                                                                                                                                 0.26*sin(theta4) + 0.12*cos(theta3)*sin(theta4) + 0.3*cos(theta5)*sin(theta4) + 0.3*cos(theta4)*sin(theta6) + 0.28*cos(theta6)*sin(theta4) + 4.2*sin(theta4)*sin(theta5) - 0.56*cos(theta5)^2*sin(theta4) + 1.68*cos(theta3)*sin(theta4)*sin(theta5) + 1.1479437019748901445007192746311e-41*cos(theta4)*sin(theta3)*sin(theta6) - 3.88*cos(theta5)*sin(theta4)*sin(theta5) - 0.56*cos(theta5)^2*cos(theta6)*sin(theta4) + 0.12*cos(theta3)*cos(theta5)*sin(theta4) + 0.12*cos(theta3)*cos(theta4)*sin(theta6) - 0.28*cos(theta4)*cos(theta5)*sin(theta6) + 0.3*cos(theta5)*cos(theta6)*sin(theta4) - 1.1479437019748901445007192746311e-41*cos(theta4)*cos(theta5)^2*sin(theta3)*sin(theta6) + 0.04*cos(theta5)*cos(theta6)^2*sin(theta4)*sin(theta5) + 0.12*cos(theta3)*cos(theta5)*cos(theta6)*sin(theta4) + 0.04*cos(theta4)*cos(theta6)*sin(theta5)*sin(theta6),                                                                                                                                                                                                                                                                                                                                                                                                                                                                                                                                                                                                                                                                                                                                                                                                                                                                                                                                                                                                                                                                                                                                                                                                                                                                                                                                                                                                                                                                                                                                                                                                                                                                                                                                                                                                                                                                                                                                                                                                                                                                                                                                                                                                                                                                                                                                                                                                                                                                                                                                                                       0.26*sin(theta4) + 0.3*cos(theta5)*sin(theta4) + 0.3*cos(theta4)*sin(theta6) + 0.28*cos(theta6)*sin(theta4) + 4.2*sin(theta4)*sin(theta5) - 0.56*cos(theta5)^2*sin(theta4) - 3.88*cos(theta5)*sin(theta4)*sin(theta5) - 0.56*cos(theta5)^2*cos(theta6)*sin(theta4) - 0.28*cos(theta4)*cos(theta5)*sin(theta6) + 0.3*cos(theta5)*cos(theta6)*sin(theta4) + 0.04*cos(theta5)*cos(theta6)^2*sin(theta4)*sin(theta5) + 0.04*cos(theta4)*cos(theta6)*sin(theta5)*sin(theta6),                                                                                                                                                                                                                                                                                                                                                                                                                                                                                                                                                                                                                                                                                                                                                                                                                                                                                                                                                                                                                                                                                                                                                                                                                                                                                                                                                                                                                                                                                                                                                                                                                                                                                                                                                                                                                                                                                                                                                                                                                                                                                                                                                                                                         0.01*cos(2.0*theta5)*cos(2.0*theta6) - 0.01*cos(2.0*theta6) - 1.9502051174171397912566328259076*cos(2.0*theta5 + 0.14407254065728860693496196531882) + 0.28*sin(2.0*theta5)*cos(theta6) + 2.0516,                                                                                                                                                                                                                                                                                                                                                                                                                                                                                                                                                                                                                                                                                                                                                                                                                                                                                                                                                                                                                                                                          -(sin(theta6)*(2.8e+71*cos(theta5) + 11479437019748901445007192746311.0*sin(theta5) - 4.0e+70*cos(theta6)*sin(theta5)))/1000000000000000000000000000000000000000000000000000000000000000000000000,                                                                                                                                                                                                                                                                                                                                                                                                                                                                                                                                                                                                                                                                                                                                                                                                                                                                             0.0401*cos(theta5) + 0.28*cos(theta6)*sin(theta5);
                                                                                                                                                                                                                                                                                                                                                                                                                                                                                                                                                                                                                                                                                                                                                                                                                                                                                                                                                                                                                                                                                                                                                                                                                                                                                                                                                                                                                                                                                                                                                                                                                                                                                                                                                                                                                                                                                                                                                                                                                                                                                                                                                                                                                                                                                                                                                                                                                                                                                                                                                                                                                                                                                                                                                                                                                                                                                                                                                                                                                                                                                                                                                                                                                                                                                                                                                                                                                                                                                                                                                                                                                                                                                                                                                                                                                                                                                                                                                                                                                                                                                                                                                                                                                                                                                                                                                                                                                                                                                                                                                                                                                                                                                                                                                                                                                                                                                                                                                                                                                                                          3.9606*sin(theta2)*sin(theta3)*sin(theta4) - 0.12*cos(theta2)*sin(theta4)*sin(theta5) - 3.9606*cos(theta2)*cos(theta3)*sin(theta4) + 1.68*cos(theta2)*cos(theta5)*sin(theta4) - 0.04*cos(theta2)*cos(theta3)*cos(theta6)^2*sin(theta4) + 0.04*cos(theta6)^2*sin(theta2)*sin(theta3)*sin(theta4) + 4.2*cos(theta2)*cos(theta3)*cos(theta5)*sin(theta4) - 0.3*cos(theta2)*cos(theta3)*sin(theta4)*sin(theta5) - 0.28*cos(theta2)*cos(theta5)*sin(theta3)*sin(theta6) - 0.28*cos(theta3)*cos(theta5)*sin(theta2)*sin(theta6) - 0.12*cos(theta2)*cos(theta6)*sin(theta4)*sin(theta5) - 4.2*cos(theta5)*sin(theta2)*sin(theta3)*sin(theta4) + 0.3*sin(theta2)*sin(theta3)*sin(theta4)*sin(theta5) - 0.28*cos(theta2)*cos(theta3)*cos(theta4)*sin(theta5)*sin(theta6) - 0.3*cos(theta2)*cos(theta3)*cos(theta6)*sin(theta4)*sin(theta5) + 0.04*cos(theta2)*cos(theta6)*sin(theta3)*sin(theta5)*sin(theta6) + 0.04*cos(theta3)*cos(theta6)*sin(theta2)*sin(theta5)*sin(theta6) + 0.28*cos(theta4)*sin(theta2)*sin(theta3)*sin(theta5)*sin(theta6) + 0.3*cos(theta6)*sin(theta2)*sin(theta3)*sin(theta4)*sin(theta5) - 0.04*cos(theta2)*cos(theta3)*cos(theta4)*cos(theta5)*cos(theta6)*sin(theta6) + 0.04*cos(theta4)*cos(theta5)*cos(theta6)*sin(theta2)*sin(theta3)*sin(theta6),                                                                                                                                                                                                                                                                                                                                                                                                                                                                                                                                                                                                                                                                                                                                                                                                                                                                                                                                                                                                                                                                                                                                                                                                                                                                                                                                                                                                                                                                                                                                                                                                                                                                                                                                                                                                                                                                                                                                                                                                                                                                                                                                                                                                                                                                                                                                                                                                                                                                                                                                                                                3.9606*cos(theta4) - 4.2*cos(theta4)*cos(theta5) + 0.12*cos(theta5)*sin(theta3) + 0.3*cos(theta4)*sin(theta5) + 1.68*sin(theta3)*sin(theta5) + 0.04*cos(theta4)*cos(theta6)^2 - 0.28*sin(theta4)*sin(theta5)*sin(theta6) - 1.68*cos(theta3)*cos(theta4)*cos(theta5) - 1.1479437019748901445007192746311e-41*cos(theta3)*cos(theta5)*cos(theta6) + 0.12*cos(theta3)*cos(theta4)*sin(theta5) + 0.12*cos(theta5)*cos(theta6)*sin(theta3) + 0.3*cos(theta4)*cos(theta6)*sin(theta5) + 0.12*cos(theta3)*cos(theta4)*cos(theta6)*sin(theta5) + 1.1479437019748901445007192746311e-41*cos(theta4)*cos(theta6)*sin(theta3)*sin(theta5) - 0.04*cos(theta5)*cos(theta6)*sin(theta4)*sin(theta6),                                                                                                                                                                                                                                                                                                                                                                                                                                                                                                                                                                                                                                                                                                                                                                                                                                                                                                                                                                                                                                                                                                                                                                                                                                                                                                                                                                                                                                                                                                                                                                                                                                                                                                                                                                                                                                                                                                                                                                                                                                                                                                                                                                                                                                                                                                                                                                                                                                                                                                                                                                                                                                                                                                                                                                                   3.9606*cos(theta4) - 4.2*cos(theta4)*cos(theta5) + 0.3*cos(theta4)*sin(theta5) + 0.04*cos(theta4)*cos(theta6)^2 - 0.28*sin(theta4)*sin(theta5)*sin(theta6) + 0.3*cos(theta4)*cos(theta6)*sin(theta5) - 0.04*cos(theta5)*cos(theta6)*sin(theta4)*sin(theta6),                                                                                                                                                                                                                                                                                                                                                                                                                                                                                                                                                                                                                                                                                                                                                                                                                                                                                                                                                                                                                                                                                                                                                                                                                                                                                                                                                                                                                                                                                                                                                                                                                                                                                                                                                                                                                                                                                                                                                                                                                                                                                                                                                                                                                                                                                                                                        -(sin(theta6)*(7.0*cos(theta5) - 1.0*cos(theta6)*sin(theta5)))/25,                                                                                                                                                                                                                                                                                                                                                                                                                                                                                                                                                                                                                                                                                                                                                                                                                                                                                                                                                                                                                                                                                                                                                                                                                                                0.04*cos(theta6)^2 + 3.9606,                                                                                                                                                                                                                                                                                                                                                                                                                                                                                                                                                                                                                                                                                                                                                                                                                                                                                                             -0.28*sin(theta6);
                                                                                                                                                                                                                                                                                                                                                                                                                                                                                                                                                                                                                                                                                                                                                                                                                                                                                                                                                                                                                                                                                                                                                                                                                                                                                                                                                                                                                                                                                                                                                                                                                                                                                                                                                                                                                                                                                                                                                                                                                                                                                                                                                                                                                                                                                                                                                                                                                                                                                                                                                                                                                                                                                                                                                                                                                                                                                                                                                                                                                                                                                                                                                                                                                                                                                                                                                                                                                                                                                                                                                                                                                                                                                                                                                                                                                                                                                                                                                                                                                                                                                                                                                                                                                                                                                                                                                                                                                                                                                                                                                                                                                                                                                                                                                                                                                                                                                                                                                                                                                                                                                                                                                                                                                                                                                                                                                                                                       0.12*cos(theta2)*cos(theta4)*cos(theta6) + 0.0401*cos(theta2)*cos(theta5)*sin(theta3) + 0.0401*cos(theta3)*cos(theta5)*sin(theta2) + 0.3*cos(theta2)*cos(theta3)*cos(theta4)*cos(theta6) + 0.0401*cos(theta2)*cos(theta3)*cos(theta4)*sin(theta5) + 0.28*cos(theta2)*cos(theta3)*sin(theta4)*sin(theta6) - 0.3*cos(theta4)*cos(theta6)*sin(theta2)*sin(theta3) + 0.28*cos(theta2)*cos(theta6)*sin(theta3)*sin(theta5) + 0.28*cos(theta3)*cos(theta6)*sin(theta2)*sin(theta5) - 0.12*cos(theta2)*cos(theta5)*sin(theta4)*sin(theta6) - 0.0401*cos(theta4)*sin(theta2)*sin(theta3)*sin(theta5) - 0.28*sin(theta2)*sin(theta3)*sin(theta4)*sin(theta6) - 0.28*cos(theta2)*cos(theta3)*cos(theta4)*cos(theta5)*cos(theta6) - 0.3*cos(theta2)*cos(theta3)*cos(theta5)*sin(theta4)*sin(theta6) + 0.28*cos(theta4)*cos(theta5)*cos(theta6)*sin(theta2)*sin(theta3) + 0.3*cos(theta5)*sin(theta2)*sin(theta3)*sin(theta4)*sin(theta6),                                                                                                                                                                                                                                                                                                                                                                                                                                                                                                                                                                                                                                                                                                                                                                                                                                                                                                                                                                                                                                                                                                                                                                                                                                                                                                                                                                                                                                                                                                                                                                                                                                                                                                                                                                                                                                                                                                                                                                                                                                                                                                                                                                                                                                                                                                                                                                                                                                                                                                                                                                                                                                                                                                                                                                                                                                                                                                                                        0.3*cos(theta6)*sin(theta4) - 0.28*cos(theta4)*sin(theta6) + 0.0401*sin(theta4)*sin(theta5) - 0.12*sin(theta3)*sin(theta5)*sin(theta6) + 0.12*cos(theta3)*cos(theta6)*sin(theta4) + 0.3*cos(theta4)*cos(theta5)*sin(theta6) - 0.28*cos(theta5)*cos(theta6)*sin(theta4) + 0.12*cos(theta3)*cos(theta4)*cos(theta5)*sin(theta6),                                                                                                                                                                                                                                                                                                                                                                                                                                                                                                                                                                                                                                                                                                                                                                                                                                                                                                                                                                                                                                                                                                                                                                                                                                                                                                                                                                                                                                                                                                                                                                                                                                                                                                                                                                                                                                                                                                                                                                                                                                                                                                                                                                                                                                                                                                                                                                                                                                                                                                                                                                                                                                                                                                                                                                                                                                                              0.3*cos(theta6)*sin(theta4) - 0.28*cos(theta4)*sin(theta6) + 0.0401*sin(theta4)*sin(theta5) + 0.3*cos(theta4)*cos(theta5)*sin(theta6) - 0.28*cos(theta5)*cos(theta6)*sin(theta4),                                                                                                                                                                                                                                                                                                                                                                                                                                                                                                                                                                                                                                                                                                                                                                                                                                                                                                                                                                                                                                                                                                                                                                                                                                                                                                                                                                                                                                                                                                                                                                                                                                                                                                                                                                                                                                                                                                                                                                                                                                                                                                                                                                                                                                                                                                                                                        0.0401*cos(theta5) + 0.28*cos(theta6)*sin(theta5),                                                                                                                                                                                                                                                                                                                                                                                                                                                                                                                                                                                                                                                                                                                                                                                                                                                                                                                                                                                                                                                                                                                                                                                                                                                          -0.28*sin(theta6),                                                                                                                                                                                                                                                                                                                                                                                                                                                                                                                                                                                                                                                                                                                                                                                                                                                                                                                        0.0401];
                                                                                                                                                                                                                                                                                                                                                                                                                                                                                                                                                                                                                                                                                                                                                                                                                                                                                                                                                                                                                                                                                                                                                                                                                                                                                                                                                                                                                                                                                                                                                                                                                                                                                                                                                                                                                                                                                                                                                                                                                                                                                                                                                                                                                                                                                                                                                                                                                                                                                                                                                                                                                                                                                                                                                                                                                                                                                                                                                                                                                                                                                                                                                                                                                                                                                                                                                                                                                                                                                                                                                                                                                                                                                                                                                                                                                                                                                                                                                                                                                                                                                                                                                                                                                                                                                                                                                                                                                                                                                                                                                                                                                                                                                                                                                                                                                                                                                                                                                                                                                                                                                                                                                                                                                                                                                                                                                                                                   
